simulink model "AutomotiveEMS"  (R2018a)
settings: Solver=VariableStepAuto  StartTime=0  StopTime=3.5  FixedStep=1e-6
undefined symbols (not defined in the file): alternator, buck, DiscIntNeverNeededParam, electrical_load, hybrid_control, i_f_max, iceToAltRotRatio, n_ice_f, n_ice_i, rectifier, t_brake_f, t_brake_i, T_k, T_r, T_s
libraries: fl_lib x43, nesl_utility x41, elec_lib x33, simulink x10, SimscapeCustomBlocks_lib x2, dsparch4 x2, pe_lib x1
(part 3 of 3)

== system AutomotiveEMS/Alternator/Armature circuit/Armature circuit (Y)/r_a ==
  Constant : Constant  Value=r_ref
  Constant1 : Constant  Value=T_ref
  Constant2 : Constant  Value=T
  Constant3 : Constant  Value=alpha
  MATLAB Function : MATLAB Function  TreatAsAtomicUnit=on
  R : fl_lib/Electrical/Electrical Elements/Variable Resistor  Rmin=0 Ohm  i_specify=off  i_priority=None  i=0 A  i_nominal_specify=off  i_nominal_unit=A  i_nominal_value=1  v_specify=off  v_priority=None  v=0 V  v_nominal_specify=off  v_nominal_unit=V  v_nominal_value=1
  Simulink-PS Converter : nesl_utility/Simulink-PS Converter  PhysicalDomain=network_engine_domain  SubClassName=ps_input  LeftPortType=input  RightPortType=output  PseudoPeriodic=off  Frequencies=[]  NoiseDistribution=none  NoiseParameters=[]  Unit=1  AffineConversion=off  FilteringAndDerivatives=provide  SimscapeFilterOrder=1  InputFilterTimeConstant=0.001  UdotUserProvided=0
  + : PMIOPort  Side=Left
  - : PMIOPort  Port=2  Side=Right
  wires:
  MATLAB Function/1(r) -> Simulink-PS Converter/1
  Constant/1 -> MATLAB Function/1(r_ref)
  Constant1/1 -> MATLAB Function/2(T_ref)
  Constant3/1 -> MATLAB Function/4(alpha)
  Constant2/1 -> MATLAB Function/3(T)
  connections:
  Simulink-PS Converter/RConn1 -- R/LConn1
  R/RConn1 -- -/RConn1
  R/LConn2 -- +/RConn1

== system AutomotiveEMS/Alternator/Armature circuit/Armature circuit (Y)/r_b ==
  Constant : Constant  Value=r_ref
  Constant1 : Constant  Value=T_ref
  Constant2 : Constant  Value=T
  Constant3 : Constant  Value=alpha
  MATLAB Function : MATLAB Function  TreatAsAtomicUnit=on
  R : fl_lib/Electrical/Electrical Elements/Variable Resistor  Rmin=0 Ohm  i_specify=off  i_priority=None  i=0 A  i_nominal_specify=off  i_nominal_unit=A  i_nominal_value=1  v_specify=off  v_priority=None  v=0 V  v_nominal_specify=off  v_nominal_unit=V  v_nominal_value=1
  Simulink-PS Converter : nesl_utility/Simulink-PS Converter  PhysicalDomain=network_engine_domain  SubClassName=ps_input  LeftPortType=input  RightPortType=output  PseudoPeriodic=off  Frequencies=[]  NoiseDistribution=none  NoiseParameters=[]  Unit=1  AffineConversion=off  FilteringAndDerivatives=provide  SimscapeFilterOrder=1  InputFilterTimeConstant=0.001  UdotUserProvided=0
  + : PMIOPort  Side=Left
  - : PMIOPort  Port=2  Side=Right
  wires:
  MATLAB Function/1(r) -> Simulink-PS Converter/1
  Constant/1 -> MATLAB Function/1(r_ref)
  Constant1/1 -> MATLAB Function/2(T_ref)
  Constant3/1 -> MATLAB Function/4(alpha)
  Constant2/1 -> MATLAB Function/3(T)
  connections:
  Simulink-PS Converter/RConn1 -- R/LConn1
  R/RConn1 -- -/RConn1
  R/LConn2 -- +/RConn1

== system AutomotiveEMS/Alternator/Armature circuit/Armature circuit (Y)/r_c ==
  Constant : Constant  Value=r_ref
  Constant1 : Constant  Value=T_ref
  Constant2 : Constant  Value=T
  Constant3 : Constant  Value=alpha
  MATLAB Function : MATLAB Function  TreatAsAtomicUnit=on
  R : fl_lib/Electrical/Electrical Elements/Variable Resistor  Rmin=0 Ohm  i_specify=off  i_priority=None  i=0 A  i_nominal_specify=off  i_nominal_unit=A  i_nominal_value=1  v_specify=off  v_priority=None  v=0 V  v_nominal_specify=off  v_nominal_unit=V  v_nominal_value=1
  Simulink-PS Converter : nesl_utility/Simulink-PS Converter  PhysicalDomain=network_engine_domain  SubClassName=ps_input  LeftPortType=input  RightPortType=output  PseudoPeriodic=off  Frequencies=[]  NoiseDistribution=none  NoiseParameters=[]  Unit=1  AffineConversion=off  FilteringAndDerivatives=provide  SimscapeFilterOrder=1  InputFilterTimeConstant=0.001  UdotUserProvided=0
  + : PMIOPort  Side=Left
  - : PMIOPort  Port=2  Side=Right
  wires:
  MATLAB Function/1(r) -> Simulink-PS Converter/1
  Constant/1 -> MATLAB Function/1(r_ref)
  Constant1/1 -> MATLAB Function/2(T_ref)
  Constant3/1 -> MATLAB Function/4(alpha)
  Constant2/1 -> MATLAB Function/3(T)
  connections:
  Simulink-PS Converter/RConn1 -- R/LConn1
  R/RConn1 -- -/RConn1
  R/LConn2 -- +/RConn1

== system AutomotiveEMS/Alternator/Armature circuit/Armature circuit (Y)/v_a sensor ==
  PS-Simulink Converter : nesl_utility/PS-Simulink Converter  PhysicalDomain=network_engine_domain  SubClassName=ps_output  LeftPortType=input  RightPortType=output  PseudoPeriodic=off  Frequencies=[]  Unit=1  AffineConversion=off
  Voltage Sensor : fl_lib/Electrical/Electrical Sensors/Voltage Sensor
  + : PMIOPort  Side=Left
  - : PMIOPort  Port=2  Side=Right
  v : Outport
  wires:
  PS-Simulink Converter/1 -> v/1
  connections:
  Voltage Sensor/LConn1 -- +/RConn1
  -/RConn1 -- Voltage Sensor/RConn2
  Voltage Sensor/RConn1 -- PS-Simulink Converter/LConn1

== system AutomotiveEMS/Alternator/Armature circuit/Armature circuit (Y)/v_b sensor ==
  PS-Simulink Converter : nesl_utility/PS-Simulink Converter  PhysicalDomain=network_engine_domain  SubClassName=ps_output  LeftPortType=input  RightPortType=output  PseudoPeriodic=off  Frequencies=[]  Unit=1  AffineConversion=off
  Voltage Sensor : fl_lib/Electrical/Electrical Sensors/Voltage Sensor
  + : PMIOPort  Side=Left
  - : PMIOPort  Port=2  Side=Right
  v : Outport
  wires:
  PS-Simulink Converter/1 -> v/1
  connections:
  Voltage Sensor/LConn1 -- +/RConn1
  -/RConn1 -- Voltage Sensor/RConn2
  Voltage Sensor/RConn1 -- PS-Simulink Converter/LConn1

== system AutomotiveEMS/Alternator/Armature circuit/Armature circuit (Y)/v_c sensor ==
  PS-Simulink Converter : nesl_utility/PS-Simulink Converter  PhysicalDomain=network_engine_domain  SubClassName=ps_output  LeftPortType=input  RightPortType=output  PseudoPeriodic=off  Frequencies=[]  Unit=1  AffineConversion=off
  Voltage Sensor : fl_lib/Electrical/Electrical Sensors/Voltage Sensor
  + : PMIOPort  Side=Left
  - : PMIOPort  Port=2  Side=Right
  v : Outport
  wires:
  PS-Simulink Converter/1 -> v/1
  connections:
  Voltage Sensor/LConn1 -- +/RConn1
  -/RConn1 -- Voltage Sensor/RConn2
  Voltage Sensor/RConn1 -- PS-Simulink Converter/LConn1

== matlab function AutomotiveEMS/Alternator/Armature circuit/Armature circuit (Delta)/r_a/MATLAB Function ==
  data: r_ref input; r output; T_ref input; T input; alpha input
function r = thermalResistance(r_ref, T_ref, T, alpha)

r = r_ref * (1 + alpha * (T - T_ref));

end

== matlab function AutomotiveEMS/Buck converter/MATLAB Function ==
  data: i_i input; v_o input; d input; eta input; v_i output; i_o output
function [v_i, i_o] = buckConverter(i_i, v_o, d, eta)

v_i = v_o/d;
i_o = i_i*(eta/d);

end

== matlab function AutomotiveEMS/Alternator/Armature circuit/Armature circuit (Delta)/r_b/MATLAB Function ==
  data: r_ref input; r output; T_ref input; T input; alpha input
function r = thermalResistance(r_ref, T_ref, T, alpha)

r = r_ref * (1 + alpha * (T - T_ref));

end

== matlab function AutomotiveEMS/Alternator/Armature circuit/Armature circuit (Y)/r_a/MATLAB Function ==
  data: r_ref input; r output; T_ref input; T input; alpha input
function r = thermalResistance(r_ref, T_ref, T, alpha)

r = r_ref * (1 + alpha * (T - T_ref));

end

== matlab function AutomotiveEMS/Alternator/Armature circuit/Armature circuit (Y)/r_b/MATLAB Function ==
  data: r_ref input; r output; T_ref input; T input; alpha input
function r = thermalResistance(r_ref, T_ref, T, alpha)

r = r_ref * (1 + alpha * (T - T_ref));

end

== matlab function AutomotiveEMS/Alternator/Armature circuit/Armature circuit (Y)/r_c/MATLAB Function ==
  data: r_ref input; r output; T_ref input; T input; alpha input
function r = thermalResistance(r_ref, T_ref, T, alpha)

r = r_ref * (1 + alpha * (T - T_ref));

end

== matlab function AutomotiveEMS/Alternator/Armature circuit/Armature circuit (Delta)/r_c/MATLAB Function ==
  data: r_ref input; r output; T_ref input; T input; alpha input
function r = thermalResistance(r_ref, T_ref, T, alpha)

r = r_ref * (1 + alpha * (T - T_ref));

end

== matlab function AutomotiveEMS/Hybrid Load Matching Controller Scheme/Hybrid Load Matching Controller/Load Matching Switched-Mode Rectifier Controller/MATLAB Function ==
  data: n_r input; u_smr output; i_f input; p input; v_o input; u_lim_l input; u_lim_u input
function u_smr = load_matching_smr_controller(n_r, i_f, p, v_o, u_lim_l, u_lim_u)

epsilon = 1e-3;

if (i_f < epsilon)
    u_smr = 0;
else
    k_e = 0;
    
    omega_r = 2*pi*n_r/60;
    omega_e = p*omega_r;
    u_smr = 1 - ((sqrt(2)*pi*k_e)/(4*v_o))*omega_e*i_f;
%     u_smr = 1 - (pi/2)*(k_e*omega_e*i_f/v_o);
    
    if (u_smr > u_lim_u)
        u_smr = u_lim_u;
    elseif (u_smr < u_lim_l)
        u_smr = u_lim_l;
    end
end

end
